simulink model "p4_individual_simulink"  (R2024b)
settings: Solver=VariableStepAuto  StartTime=0  StopTime=500  FixedStep=.1  RelTol=1e-3
values from neighbouring files (symbols this model uses):
  C0 = 0.0041    [p4_indiviual_init_cons.m]
  C1 = 0.000066    (= 6.6e-05)    [p4_indiviual_init_cons.m]
  C2 = 0.5*Rho*A*Cd    (= 0.5733)    [p4_indiviual_init_cons.m]
  efficency = .95    (= 0.95)    [p4_indiviual_init_cons.m]
undefined symbols (not defined in the file or in its folder): carData, datBat, datMotor
settings Model: Creator=Jake Sanders  LastModifiedBy=Jake Sanders

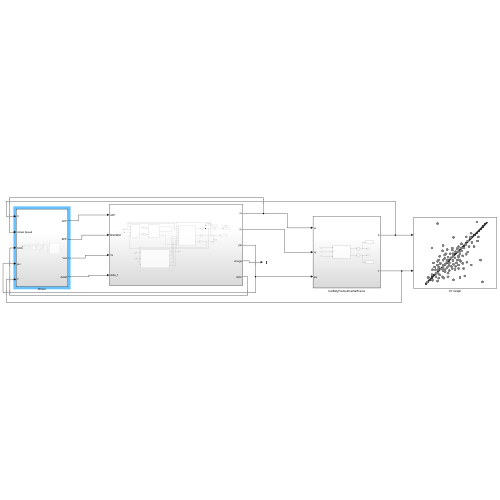
[thumbnail: Simulink's stored preview of the top-level diagram]
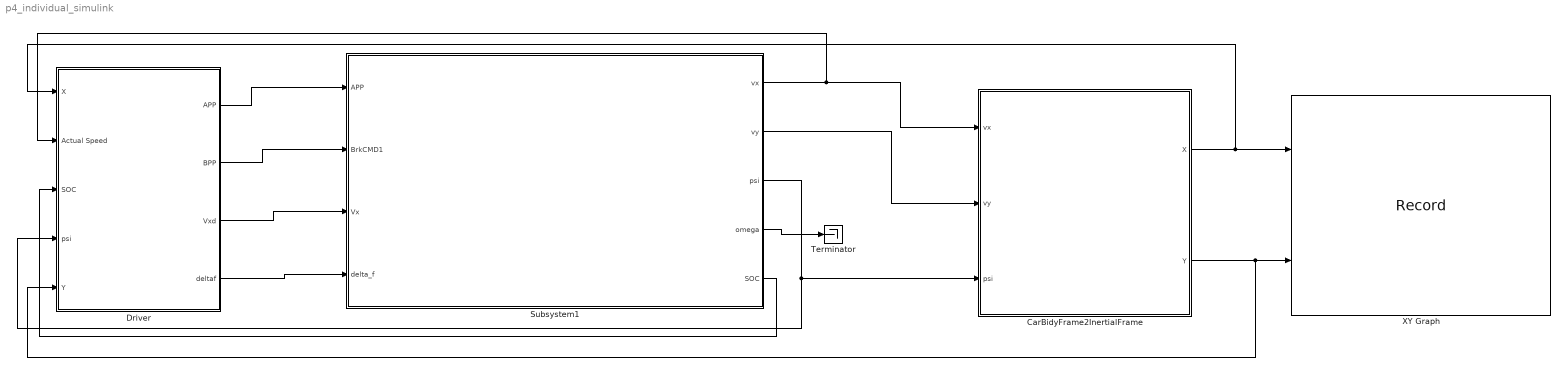
== system p4_individual_simulink ==
  CarBidyFrame2InertialFrame : Subsystem
  Driver : Subsystem
  Subsystem1 : Subsystem
  Terminator : Terminator
  XY Graph : Record  FileSettingsInternal="{\"entries\":[{\"content\":{\"excelSettings\":{\"content\":{},\"type\":\"Streamout.ExcelSettings\"}},\"type\":\"Streamout.FileSettingStorage\",\"uuid\":\"\"}],\"packageUris\":[\"http:\\/\\/schema.mathworks.com\\/mf0\\/streamout_blocks\\/R2020a\"],\"version\":\"1.0\"}"  Layout=[1 1]  SignalsInternal="{\"entries\":[{\"content\":{\"signals\":[{\"content\":{\"blockPath\":[],\"dimensions\":[1],\"domain\":\"\",\"lineColor\":\"#a2142f\",\"plots\":[ 1 ],\"port\":1,\"sid\":[\"\"],\"signalID\":1,\"signalName\":\"CarBidyFrame2InertialFrame:1\"},\"type\":\"RecordBlkView.Signal\",\"uuid\":\"\"},{\"content\":{\"blockPath\":[],\"dimensions\":[1],\"domain\":\"\",\"lineColor\":\"#139fff\",\"plots\":[ 1 ],\"port\":2,\"sid\":[\"\"],\"signalID\":2,\"signalName\":\"CarBidyFrame2InertialFrame:2\"},\"type\":\"RecordBlkView.Signal\",\"uuid\":\"\"},{\"content\":{\"blockPath\":[],\"dimensions\":[1],\"domain\":\"\",\"lineColor\":\"#ff6929\",\"lineWidth\":2,\"port\":1,\"sid\":[\"\"],\"signalID\":3,\"signalName\":\"Integrator\"},\"type\":\"RecordBlkView.Signal\",\"uuid\":\"\"},{\"content\":{\"blockPath\":[],\"dimensions\":[1],\"domain\":\"\",\"lineColor\":\"#b746ff\",\"lineWidth\":2,\"port\":1,\"sid\":[\"\"],\"signalID\":4,\"signalName\":\"Integrator1\"},\"type\":\"RecordBlkView.Signal\",\"uuid\":\"\"},{\"content\":{\"blockPath\":[],\"dimensions\":[1],\"domain\":\"\",\"lineColor\":\"#64d413\",\"lineWidth\":2,\"port\":1,\"sid\":[\"\"],\"signalID\":5,\"signalName\":\"MATLAB Function3\"},\"type\":\"RecordBlkView.Signal\",\"uuid\":\"\"},{\"content\":{\"blockPath\":[],\"dimensions\":[1],\"domain\":\"\",\"lineColor\":\"#ff13a6\",\"lineWidth\":2,\"port\":1,\"sid\":[\"\"],\"signalID\":6,\"signalName\":\"MATLAB Function5\"},\"type\":\"RecordBlkView.Signal\",\"uuid\":\"\"},{\"content\":{\"blockPath\":[],\"dimensions\":[1],\"domain\":\"\",\"lineColor\":\"#fe330a\",\"lineWidth\":2,\"port\":1,\"sid\":[\"\"],\"signalID\":7,\"signalName\":\"Integrator\"},\"type\":\"RecordBlkView.Signal\",\"uuid\":\"\"},{\"content\":{\"blockPath\":[],\"dimensions\":[1],\"domain\":\"\",\"lineColor\":\"#22b573\",\"lineWidth\":2,\"port\":1,\"sid\":[\"\"],\"signalID\":8,\"signalName\":\"Integrator1\"},\"type\":\"RecordBlkView.Signal\",\"uuid\":\"\"},{\"content\":{\"blockPath\":[],\"dimensions\":[1],\"domain\":\"\",\"lineColor\":\"#0072bd\",\"lineWidth\":2,\"port\":1,\"sid\":[\"\"],\"signalID\":9,\"signalName\":\"Integrator2\"},\"type\":\"RecordBlkView.Signal\",\"uuid\":\"\"},{\"content\":{\"blockPath\":[],\"dimensions\":[1],\"domain\":\"\",\"lineColor\":\"#d95319\",\"lineWidth\":2,\"port\":1,\"sid\":[\"\"],\"signalID\":10,\"signalName\":\"drag forces\"},\"type\":\"RecordBlkView.Signal\",\"uuid\":\"\"},{\"content\":{\"blockPath\":[],\"dimensions\":[1],\"domain\":\"\",\"lineColor\":\"#edb120\",\"lineWidth\":2,\"port\":1,\"sid\":[\"\"],\"signalID\":11,\"signalName\":\"Electric Motor Drve:3\"},\"type\":\"RecordBlkView.Signal\",\"uuid\":\"\"},{\"content\":{\"blockPath\":[],\"dimensions\":[1],\"domain\":\"\",\"lineColor\":\"#7e2f8e\",\"lineWidth\":2,\"port\":1,\"sid\":[\"\"],\"signalID\":12,\"signalName\":\"Gain5\"},\"type\":\"RecordBlkView.Signal\",\"uuid\":\"\"},{\"content\":{\"blockPath\":[],\"dimensions\":[1],\"domain\":\"\",\"lineColor\":\"#77ac30\",\"lineWidth\":2,\"port\":1,\"sid\":[\"\"],\"signalID\":13,\"signalName\":\"Integrator1\"},\"type\":\"RecordBlkView.Signal\",\"uuid\":\"\"},{\"content\":{\"blockPath\":[],\"dimensions\":[1],\"domain\":\"\",\"lineColor\":\"#4dbeee\",\"lineWidth\":2,\"port\":1,\"sid\":[\"\"],\"signalID\":14,\"signalName\":\"1-D Lookup\\nTable\"},\"type\":\"RecordBlkView.Signal\",\"uuid\":\"\"},{\"content\":{\"blockPath\":[],\"dimensions\":[1],\"domain\":\"\",\"lineColor\":\"#a2142f\",\"lineWidth\":2,\"port\":1,\"sid\":[\"\"],\"signalID\":15,\"signalName\":\"Motor Efficiency Table\"},\"type\":\"RecordBlkView.Signal\",\"uuid\":\"\"},{\"content\":{\"blockPath\":[],\"dimensions\":[1],\"domain\":\"\",\"lineColor\":\"#139fff\",\"lineWidth\":2,\"port\":1,\"sid\":[\"\"],\"signalID\":16,\"signalName\":\"Product1\"},\"type\":\"RecordBlkView.Signal\",\"uuid\":\"\"},{\"content\":{\"blockPath\":[],\"dimensions\":[1],\"domain\":\"\",\"lineColor\":\"#ff6929\",\"lineWidth\":2,\"port\":1,\"sid\":[\"\"],\"signalID\":17,\"signalName\":\"Integrator\"},\"type\":\"RecordBlkView.Signal\",\"uuid\":\"\"},{\"content\":{\"blockPath\":[],\"dimensions\":[1],\"domain\":\"\",\"lineColor\":\"#b746ff\",\"lineWidth\":2,\"port\":1,\"sid\":[\"\"],\"signalID\":18,\"signalName\":\"Bus Voltage\"},\"type\":\"RecordBlkView.Signal\",\"uuid\":\"\"},{\"content\":{\"blockPath\":[],\"dimensions\":[1],\"domain\":\"\",\"lineColor\":\"#64d413\",\"lineWidth\":2,\"port\":1,\"sid\":[\"\"],\"signalID\":19,\"signalName\":\"Unit Delay\"},\"type\":\"RecordBlkView.Signal\",\"uuid\":\"\"},{\"content\":{\"blockPath\":[],\"dimensions\":[1],\"domain\":\"\",\"lineColor\":\"#ff13a6\",\"lineWidth\":2,\"port\":1,\"sid\":[\"\"],\"signalID\":20,\"signalName\":\"MATLAB Function:2\"},\"type\":\"RecordBlkView.Signal\",\"uuid\":\"\"}]},\"type\":\"RecordBlkView.InputSignals\",\"uuid\":\"\"}],\"packageUris\":[\"http:\\/\\/schema.mathworks.com\\/mf0\\/streamout_blocks\\/R2020a\"],\"version\":\"1.0\"}"  VisualizationBindings="{\"xyplotplugin\":{\"info\":[{\"series\":[{\"bindingParametersList\":[{\"parameter\":\"X-Axis\",\"signalID\":1,\"signalName\":\"CarBidyFrame2InertialFrame:1\"},{\"parameter\":\"Y-Axis\",\"signalID\":2,\"signalName\":\"CarBidyFrame2InertialFrame:2\"}],\"seriesID\":0}],\"subplotID\":1}]}}"  CompatibilityTag=XY
  wires:
  CarBidyFrame2InertialFrame/2(Y) -> Driver/5(Y), XY Graph/2
  CarBidyFrame2InertialFrame/1(X) -> Driver/1(X), XY Graph/1
  Driver/1(APP) -> Subsystem1/1(APP)
  Driver/2(BPP) -> Subsystem1/2(BrkCMD1)
  Driver/3(Vxd) -> Subsystem1/3(Vx)
  Driver/4(deltaf) -> Subsystem1/4(delta_f)
  Subsystem1/5(SOC) -> Driver/3(SOC)
  Subsystem1/3(psi) -> Driver/4(psi), CarBidyFrame2InertialFrame/3(psi)
  Subsystem1/2(vy) -> CarBidyFrame2InertialFrame/2(vy)
  Subsystem1/1(vx) -> Driver/2(Actual Speed), CarBidyFrame2InertialFrame/1(vx)
  Subsystem1/4(omega) -> Terminator/1

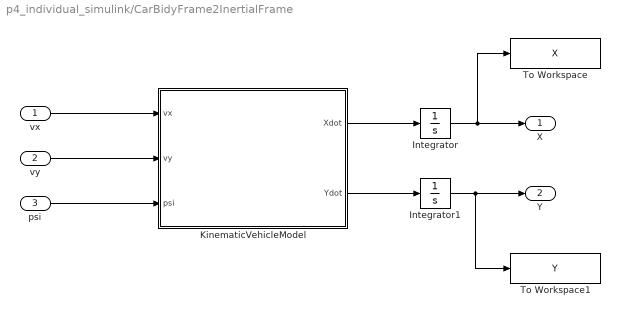
== system p4_individual_simulink/CarBidyFrame2InertialFrame ==
  vx : Inport
  vy : Inport  Port=2
  psi : Inport  Port=3
  Integrator : Integrator  InitialCondition=carData.init.X0
  Integrator1 : Integrator  InitialCondition=carData.init.Y0
  KinematicVehicleModel : MATLAB Function  TreatAsAtomicUnit=on
  To Workspace : ToWorkspace  VariableName=X  SaveFormat=Timeseries  SampleTime=.5
  To Workspace1 : ToWorkspace  VariableName=Y  SaveFormat=Timeseries  SampleTime=.5
  X : Outport
  Y : Outport  Port=2
  wires:
  vy/1 -> KinematicVehicleModel/2(vy)
  vx/1 -> KinematicVehicleModel/1(vx)
  psi/1 -> KinematicVehicleModel/3(psi)
  KinematicVehicleModel/1(Xdot) -> Integrator/1
  KinematicVehicleModel/2(Ydot) -> Integrator1/1
  Integrator/1 -> To Workspace/1, X/1
  Integrator1/1 -> To Workspace1/1, Y/1

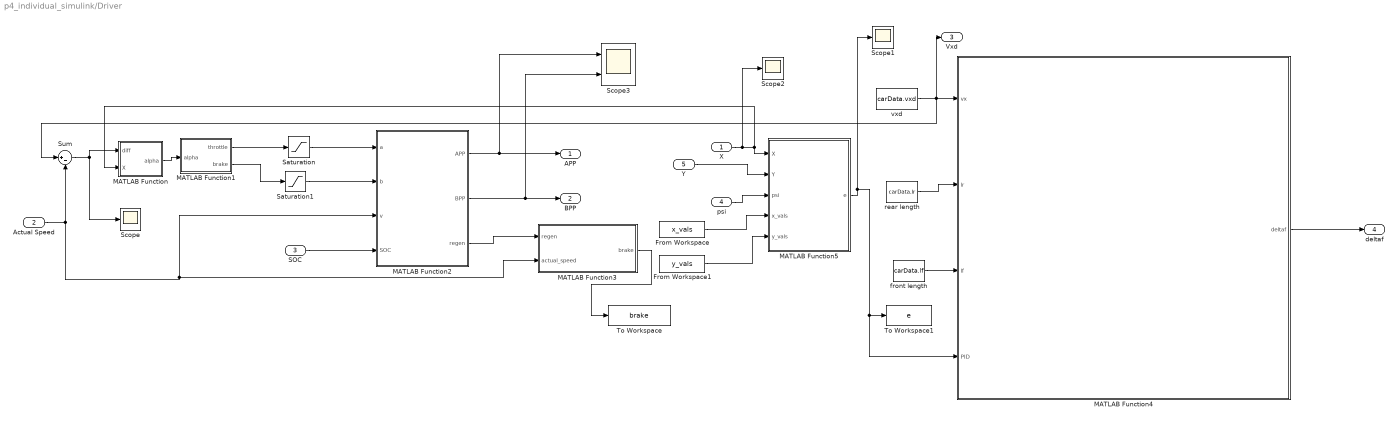
== system p4_individual_simulink/Driver ==
  X : Inport
  Actual Speed : Inport  Port=2
  SOC : Inport  Port=3
  psi : Inport  Port=4
  Y : Inport  Port=5
  From Workspace : FromWorkspace  VariableName=x_vals
  From Workspace1 : FromWorkspace  VariableName=y_vals
  MATLAB Function : MATLAB Function  TreatAsAtomicUnit=on
  MATLAB Function1 : MATLAB Function  TreatAsAtomicUnit=on
  MATLAB Function2 : MATLAB Function  TreatAsAtomicUnit=on
  MATLAB Function3 : MATLAB Function  TreatAsAtomicUnit=on
  MATLAB Function4 : MATLAB Function  TreatAsAtomicUnit=on
  MATLAB Function5 : MATLAB Function  TreatAsAtomicUnit=on
  Saturation : Saturate  UpperLimit=1  LowerLimit=0
  Saturation1 : Saturate  UpperLimit=0  LowerLimit=-1
  Scope : Scope
  Scope1 : Scope
  Scope2 : Scope
  Scope3 : Scope  NumInputPorts=2
  Sum : Sum  Inputs=|+-
  To Workspace : ToWorkspace  VariableName=brake  SaveFormat=Timeseries  SampleTime=-1
  To Workspace1 : ToWorkspace  VariableName=e  SaveFormat=Timeseries  SampleTime=-1
  front length : Constant  Value=carData.lf
  rear length : Constant  Value=carData.lr
  vxd : Constant  Value=carData.vxd
  APP : Outport
  BPP : Outport  Port=2
  Vxd : Outport  Port=3
  deltaf : Outport  Port=4
  wires:
  Actual Speed/1 -> Sum/2, MATLAB Function2/3(v), MATLAB Function3/2(actual_speed)
  MATLAB Function/1(alpha) -> MATLAB Function1/1(alpha)
  Sum/1 -> Scope/1, MATLAB Function/1(diff)
  Saturation/1 -> MATLAB Function2/1(a)
  MATLAB Function2/2(BPP) -> Scope3/2, BPP/1
  MATLAB Function1/1(throttle) -> Saturation/1
  MATLAB Function2/1(APP) -> Scope3/1, APP/1
  MATLAB Function2/3(regen) -> MATLAB Function3/1(regen)
  MATLAB Function3/1(brake) -> To Workspace/1
  MATLAB Function1/2(brake) -> Saturation1/1
  Saturation1/1 -> MATLAB Function2/2(b)
  SOC/1 -> MATLAB Function2/4(SOC)
  X/1 -> Scope2/1, MATLAB Function5/1(X), MATLAB Function/2(X)
  MATLAB Function5/1(e) -> Scope1/1, MATLAB Function4/4(PID), To Workspace1/1
  Y/1 -> MATLAB Function5/2(Y)
  front length/1 -> MATLAB Function4/3(lf)
  psi/1 -> MATLAB Function5/3(psi)
  vxd/1 -> Sum/1, Vxd/1, MATLAB Function4/1(vx)
  rear length/1 -> MATLAB Function4/2(lr)
  MATLAB Function4/1(deltaf) -> deltaf/1
  From Workspace/1 -> MATLAB Function5/4(x_vals)
  From Workspace1/1 -> MATLAB Function5/5(y_vals)

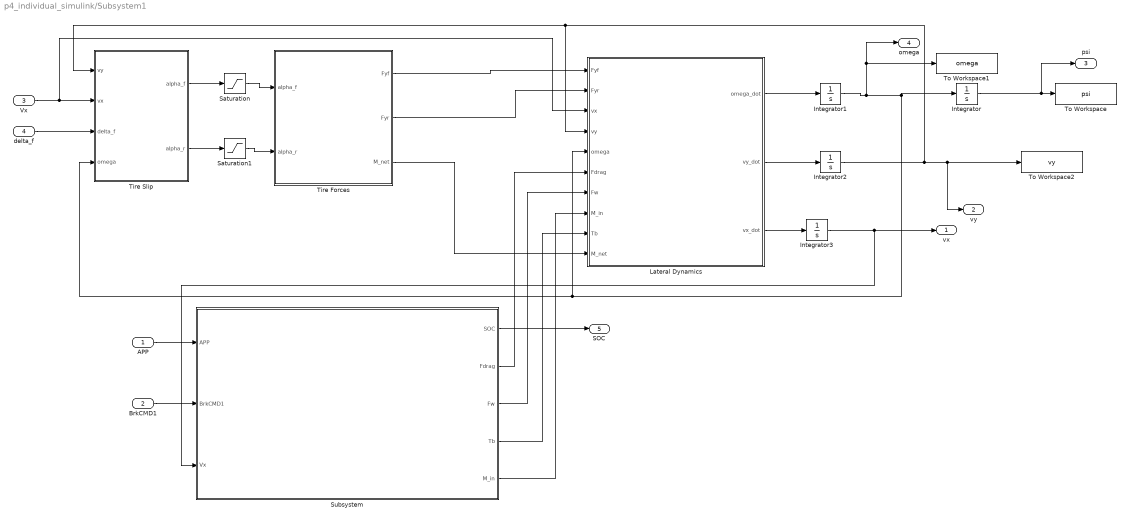
== system p4_individual_simulink/Subsystem1 ==
  APP : Inport
  BrkCMD1 : Inport  Port=2
  Vx : Inport  Port=3
  delta_f : Inport  Port=4
  " Tire Slip" : MATLAB Function  TreatAsAtomicUnit=on
  Integrator : Integrator  InitialCondition=carData.init.psi0
  Integrator1 : Integrator  InitialCondition=carData.init.omega0
  Integrator2 : Integrator  InitialCondition=carData.init.vy0
  Integrator3 : Integrator
  Lateral Dynamics : MATLAB Function  TreatAsAtomicUnit=on
  Saturation : Saturate
  Saturation1 : Saturate
  Subsystem : Subsystem
  Tire Forces : MATLAB Function  TreatAsAtomicUnit=on
  To Workspace : ToWorkspace  VariableName=psi  SaveFormat=Timeseries  SampleTime=.5
  To Workspace1 : ToWorkspace  VariableName=omega  SaveFormat=Timeseries  SampleTime=-1
  To Workspace2 : ToWorkspace  VariableName=vy  SaveFormat=Timeseries  SampleTime=-1
  vx : Outport
  vy : Outport  Port=2
  psi : Outport  Port=3
  omega : Outport  Port=4
  SOC : Outport  Port=5
  wires:
  APP/1 -> Subsystem/1(APP)
  BrkCMD1/1 -> Subsystem/2(BrkCMD1)
  Subsystem/1(SOC) -> SOC/1
  Lateral Dynamics/1(omega_dot) -> Integrator1/1
  Integrator2/1 -> Lateral Dynamics/4(vy), " Tire Slip"/1(vy), To Workspace2/1, vy/1
  Integrator1/1 -> Lateral Dynamics/5(omega), " Tire Slip"/4(omega), Integrator/1, omega/1, To Workspace1/1
  Saturation/1 -> Tire Forces/1(alpha_f)
  Tire Forces/1(Fyf) -> Lateral Dynamics/1(Fyf)
  Saturation1/1 -> Tire Forces/2(alpha_r)
  delta_f/1 -> " Tire Slip"/3(delta_f)
  Lateral Dynamics/2(vy_dot) -> Integrator2/1
  " Tire Slip"/1(alpha_f) -> Saturation/1
  Integrator/1 -> psi/1, To Workspace/1
  " Tire Slip"/2(alpha_r) -> Saturation1/1
  Tire Forces/2(Fyr) -> Lateral Dynamics/2(Fyr)
  Vx/1 -> Lateral Dynamics/3(vx), " Tire Slip"/2(vx)
  Tire Forces/3(M_net) -> Lateral Dynamics/10(M_net)
  Subsystem/2(Fdrag) -> Lateral Dynamics/6(Fdrag)
  Subsystem/3(Fw) -> Lateral Dynamics/7(Fw)
  Subsystem/4(Tb) -> Lateral Dynamics/9(Tb)
  Subsystem/5(M_in) -> Lateral Dynamics/8(M_in)
  Lateral Dynamics/3(vx_dot) -> Integrator3/1
  Integrator3/1 -> Subsystem/3(Vx), vx/1

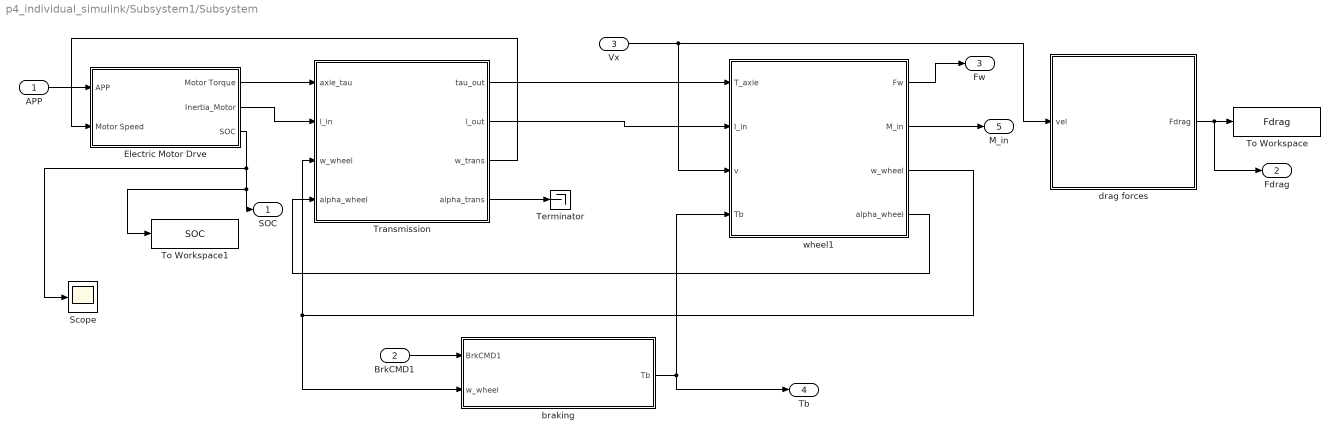
== system p4_individual_simulink/Subsystem1/Subsystem ==
  APP : Inport
  BrkCMD1 : Inport  Port=2
  Vx : Inport  Port=3
  Electric Motor Drve : Subsystem
  Scope : Scope
  Terminator : Terminator
  To Workspace : ToWorkspace  VariableName=Fdrag  SaveFormat=Timeseries  SampleTime=-1
  To Workspace1 : ToWorkspace  VariableName=SOC  SaveFormat=Timeseries  SampleTime=-1
  Transmission : Subsystem
  braking : Subsystem
  drag forces : Subsystem
  wheel1 : Subsystem
  SOC : Outport
  Fdrag : Outport  Port=2
  Fw : Outport  Port=3
  Tb : Outport  Port=4
  M_in : Outport  Port=5
  wires:
  Transmission/1(tau_out) -> wheel1/1(T_axle)
  Transmission/3(w_trans) -> Electric Motor Drve/2(Motor Speed)
  wheel1/4(alpha_wheel) -> Transmission/4(alpha_wheel)
  Electric Motor Drve/2(Inertia_Motor) -> Transmission/2(l_in)
  Electric Motor Drve/1(Motor Torque) -> Transmission/1(axle_tau)
  wheel1/3(w_wheel) -> Transmission/3(w_wheel), braking/2(w_wheel)
  Electric Motor Drve/3(SOC) -> Scope/1, To Workspace1/1, SOC/1
  APP/1 -> Electric Motor Drve/1(APP)
  BrkCMD1/1 -> braking/1(BrkCMD1)
  drag forces/1(Fdrag) -> Fdrag/1, To Workspace/1
  wheel1/1(Fw) -> Fw/1
  braking/1(Tb) -> wheel1/4(Tb), Tb/1
  Vx/1 -> wheel1/3(v), drag forces/1(vel)
  wheel1/2(M_in) -> M_in/1
  Transmission/2(l_out) -> wheel1/2(I_in)
  Transmission/4(alpha_trans) -> Terminator/1

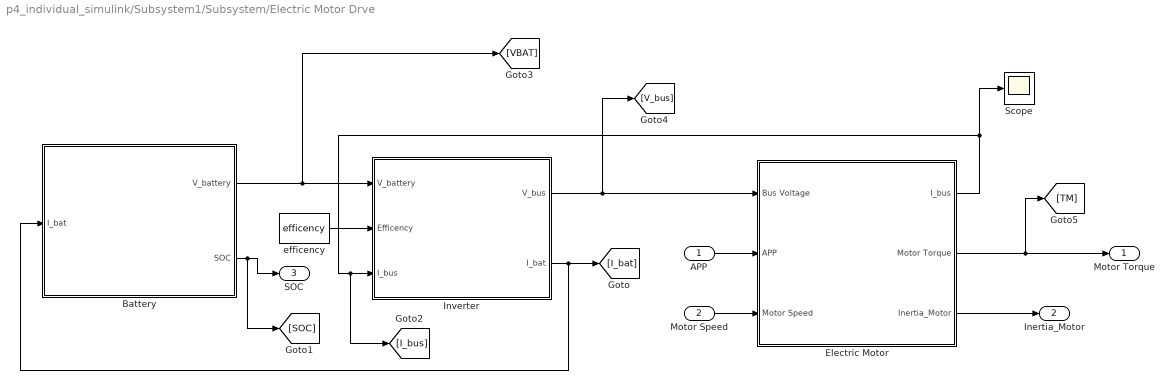
== system p4_individual_simulink/Subsystem1/Subsystem/Electric Motor Drve ==
  APP : Inport
  Motor Speed : Inport  Port=2
  Battery : Subsystem
  Electric Motor : Subsystem
  Inverter : Subsystem
  Scope : Scope
  efficency : Constant  Value=efficency
  Motor Torque : Outport
  Inertia_Motor : Outport  Port=2
  SOC : Outport  Port=3
  wires:
  Inverter/1(V_bus) -> [V_bus], Electric Motor/1(Bus Voltage)
  Inverter/2(I_bat) -> Battery/1(I_bat), [I_bat]
  Electric Motor/1(I_bus) -> Scope/1, [I_bus], Inverter/3(I_bus)
  Electric Motor/2(Motor Torque) -> [TM], Motor Torque/1
  Electric Motor/3(Inertia_Motor) -> Inertia_Motor/1
  APP/1 -> Electric Motor/2(APP)
  Motor Speed/1 -> Electric Motor/3(Motor Speed)
  efficency/1 -> Inverter/2(Efficency)
  Battery/1(V_battery) -> [VBAT], Inverter/1(V_battery)
  Battery/2(SOC) -> [SOC], SOC/1

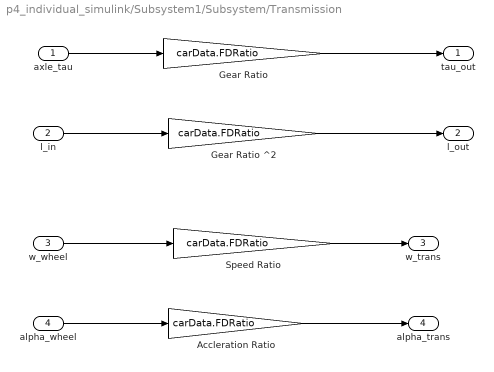
== system p4_individual_simulink/Subsystem1/Subsystem/Transmission ==
  axle_tau : Inport
  l_in : Inport  Port=2
  w_wheel : Inport  Port=3
  alpha_wheel : Inport  Port=4
  Accleration Ratio : Gain  Gain=carData.FDRatio
  Gear Ratio : Gain  Gain=carData.FDRatio
  Gear Ratio ^2 : Gain  Gain=carData.FDRatio
  Speed Ratio : Gain  Gain=carData.FDRatio
  tau_out : Outport
  l_out : Outport  Port=2
  w_trans : Outport  Port=3
  alpha_trans : Outport  Port=4
  wires:
  axle_tau/1 -> Gear Ratio/1
  Gear Ratio/1 -> tau_out/1
  w_wheel/1 -> Speed Ratio/1
  Speed Ratio/1 -> w_trans/1
  alpha_wheel/1 -> Accleration Ratio/1
  Accleration Ratio/1 -> alpha_trans/1
  l_in/1 -> Gear Ratio ^2/1
  Gear Ratio ^2/1 -> l_out/1

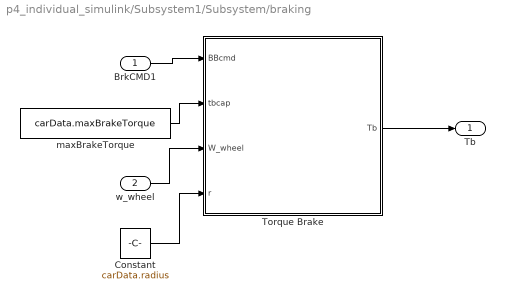
== system p4_individual_simulink/Subsystem1/Subsystem/braking ==
  BrkCMD1 : Inport
  w_wheel : Inport  Port=2
  Constant : Constant  Value=carData.radius
  Torque Brake : MATLAB Function  TreatAsAtomicUnit=on
  maxBrakeTorque : Constant  Value=carData.maxBrakeTorque
  Tb : Outport
  wires:
  w_wheel/1 -> Torque Brake/3(W_wheel)
  maxBrakeTorque/1 -> Torque Brake/2(tbcap)
  Torque Brake/1(Tb) -> Tb/1
  BrkCMD1/1 -> Torque Brake/1(BBcmd)
  Constant/1 -> Torque Brake/4(r)

== system p4_individual_simulink/Subsystem1/Subsystem/drag forces ==
  vel : Inport
  C0 : Constant  Value=C0
  C1 : Constant  Value=C1
  C2 : Constant  Value=C2
  MATLAB Function1 : MATLAB Function  TreatAsAtomicUnit=on
  Fdrag : Outport
  wires:
  vel/1 -> MATLAB Function1/1(vel)
  C0/1 -> MATLAB Function1/2(C0)
  C1/1 -> MATLAB Function1/3(C1)
  C2/1 -> MATLAB Function1/4(C2)
  MATLAB Function1/1(Fdrag) -> Fdrag/1

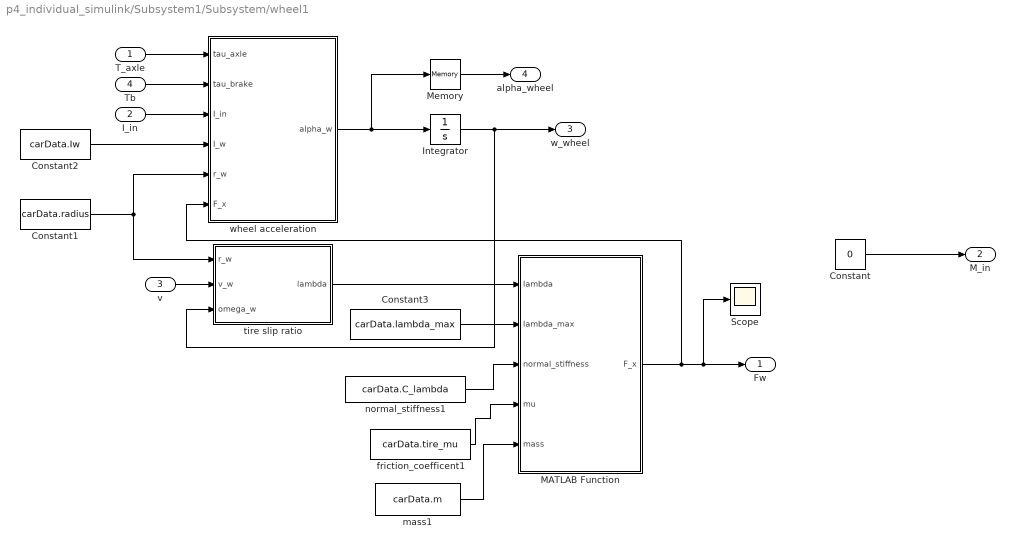
== system p4_individual_simulink/Subsystem1/Subsystem/wheel1 ==
  T_axle : Inport
  I_in : Inport  Port=2
  v : Inport  Port=3
  Tb : Inport  Port=4
  Constant : Constant  Value=0
  Constant1 : Constant  Value=carData.radius
  Constant2 : Constant  Value=carData.Iw
  Constant3 : Constant  Value=carData.lambda_max
  Integrator : Integrator
  MATLAB Function : MATLAB Function  TreatAsAtomicUnit=on
  Memory : Memory
  Scope : Scope
  friction_coefficent1 : Constant  Value=carData.tire_mu
  mass1 : Constant  Value=carData.m
  normal_stiffness1 : Constant  Value=carData.C_lambda
  tire slip ratio : MATLAB Function  TreatAsAtomicUnit=on
  wheel acceleration : MATLAB Function  TreatAsAtomicUnit=on
  Fw : Outport
  M_in : Outport  Port=2
  w_wheel : Outport  Port=3
  alpha_wheel : Outport  Port=4
  wires:
  MATLAB Function/1(F_x) -> wheel acceleration/6(F_x), Scope/1, Fw/1
  normal_stiffness1/1 -> MATLAB Function/3(normal_stiffness)
  friction_coefficent1/1 -> MATLAB Function/4(mu)
  mass1/1 -> MATLAB Function/5(mass)
  Constant3/1 -> MATLAB Function/2(lambda_max)
  tire slip ratio/1(lambda) -> MATLAB Function/1(lambda)
  Constant/1 -> M_in/1
  Memory/1 -> alpha_wheel/1
  wheel acceleration/1(alpha_w) -> Integrator/1, Memory/1
  Constant1/1 -> tire slip ratio/1(r_w), wheel acceleration/5(r_w)
  Constant2/1 -> wheel acceleration/4(I_w)
  I_in/1 -> wheel acceleration/3(I_in)
  Tb/1 -> wheel acceleration/2(tau_brake)
  T_axle/1 -> wheel acceleration/1(tau_axle)
  Integrator/1 -> w_wheel/1, tire slip ratio/3(omega_w)
  v/1 -> tire slip ratio/2(v_w)

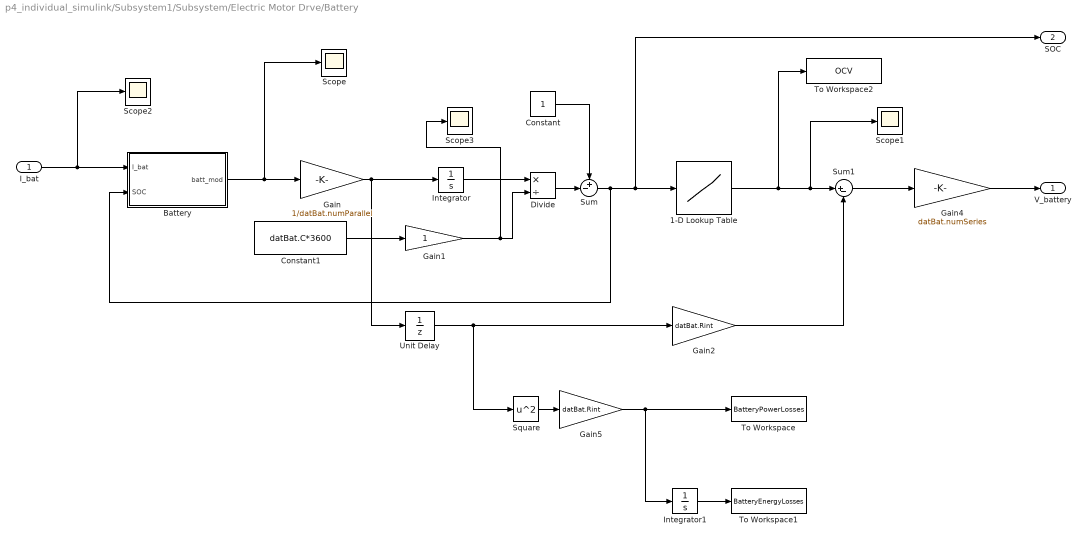
== system p4_individual_simulink/Subsystem1/Subsystem/Electric Motor Drve/Battery ==
  I_bat : Inport
  1-D Lookup Table : Lookup_n-D  NumberOfTableDimensions=1  BreakpointsForDimension1=datBat.SOC  Table=datBat.OCV  InternalRulePriority=Speed  RndMeth=Simplest
  Battery : MATLAB Function  TreatAsAtomicUnit=on
  Constant : Constant
  Constant1 : Constant  Value=datBat.C*3600
  Divide : Product  Inputs=*/
  Gain : Gain  Gain=1/datBat.numParallel
  Gain1 : Gain
  Gain2 : Gain  Gain=datBat.Rint
  Gain4 : Gain  Gain=datBat.numSeries
  Gain5 : Gain  Gain=datBat.Rint
  Integrator : Integrator
  Integrator1 : Integrator
  Scope{,1..3} (4 alike) : Scope
  Square : Math  Operator=square
  Sum : Sum  Inputs=+-|
  Sum1 : Sum  Inputs=|+-
  To Workspace : ToWorkspace  VariableName=BatteryPowerLosses  SaveFormat=Timeseries  SampleTime=-1
  To Workspace1 : ToWorkspace  VariableName=BatteryEnergyLosses  SaveFormat=Timeseries  SampleTime=-1
  To Workspace2 : ToWorkspace  VariableName=OCV  SaveFormat=Timeseries  SampleTime=-1
  Unit Delay : UnitDelay  SampleTime=-1  HasFrameUpgradeWarning=on
  V_battery : Outport
  SOC : Outport  Port=2
  wires:
  Gain5/1 -> Integrator1/1, To Workspace/1
  Integrator/1 -> Divide/1
  1-D Lookup Table/1 -> To Workspace2/1, Scope1/1, Sum1/1
  Sum1/1 -> Gain4/1
  Gain2/1 -> Sum1/2
  Battery/1(batt_mod) -> Scope/1, Gain/1
  Sum/1 -> Battery/2(SOC), SOC/1, 1-D Lookup Table/1
  Unit Delay/1 -> Square/1, Gain2/1
  Constant/1 -> Sum/1
  Divide/1 -> Sum/2
  Constant1/1 -> Gain1/1
  Integrator1/1 -> To Workspace1/1
  Gain4/1 -> V_battery/1
  Square/1 -> Gain5/1
  Gain1/1 -> Scope3/1, Divide/2
  I_bat/1 -> Scope2/1, Battery/1(I_bat)
  Gain/1 -> Unit Delay/1, Integrator/1

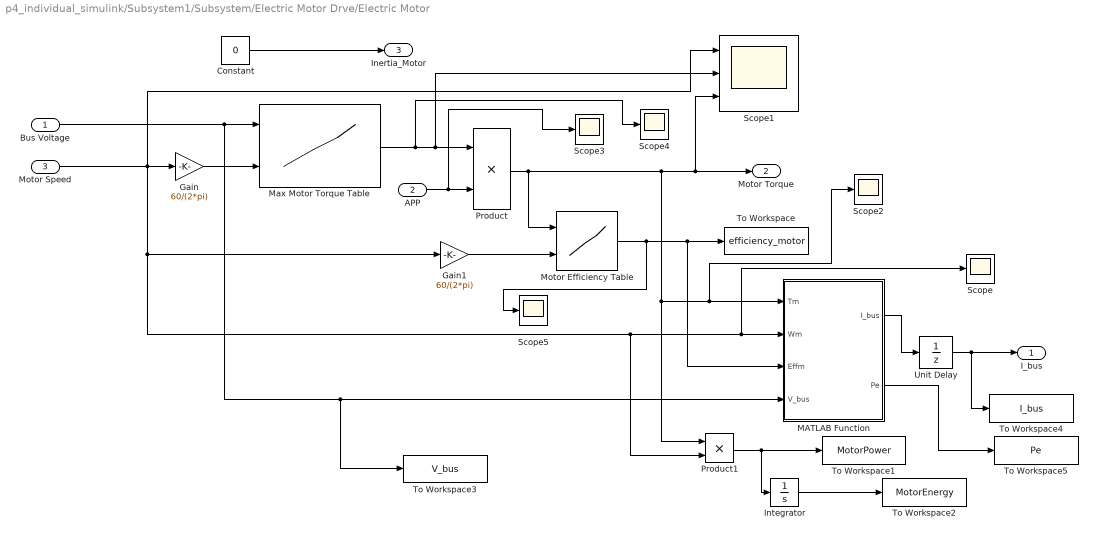
== system p4_individual_simulink/Subsystem1/Subsystem/Electric Motor Drve/Electric Motor ==
  Bus Voltage : Inport
  APP : Inport  Port=2
  Motor Speed : Inport  Port=3
  Constant : Constant  Value=0
  Gain : Gain  Gain=60/(2*pi)
  Gain1 : Gain  Gain=60/(2*pi)
  Integrator : Integrator
  MATLAB Function : MATLAB Function  TreatAsAtomicUnit=on
  "Max Motor Torque Table " : Lookup_n-D  BreakpointsForDimension1=datMotor.vbus  BreakpointsForDimension2=datMotor.rpm  Table=datMotor.maxtorque  InternalRulePriority=Speed  RndMeth=Simplest
      settings: InputPortMap=u0,u1
  Motor Efficiency Table : Lookup_n-D  BreakpointsForDimension1=datMotor.eta_torque  BreakpointsForDimension2=datMotor.eta_speed  Table=datMotor.eta_val  InternalRulePriority=Speed  RndMeth=Simplest
      settings: InputPortMap=u0,u1
  Product : Product
  Product1 : Product
  Scope{,2..5} (5 alike) : Scope
  Scope1 : Scope  NumInputPorts=3
  To Workspace : ToWorkspace  VariableName=efficiency_motor  SaveFormat=Timeseries  SampleTime=-1
  To Workspace1 : ToWorkspace  VariableName=MotorPower  SaveFormat=Timeseries  SampleTime=-1
  To Workspace2 : ToWorkspace  VariableName=MotorEnergy  SaveFormat=Timeseries  SampleTime=.5
  To Workspace3 : ToWorkspace  VariableName=V_bus  SaveFormat=Timeseries  SampleTime=-1
  To Workspace4 : ToWorkspace  VariableName=I_bus  SaveFormat=Timeseries  SampleTime=-1
  To Workspace5 : ToWorkspace  VariableName=Pe  SaveFormat=Timeseries  SampleTime=-1
  Unit Delay : UnitDelay  SampleTime=-1  HasFrameUpgradeWarning=on
  I_bus : Outport
  Motor Torque : Outport  Port=2
  Inertia_Motor : Outport  Port=3
  wires:
  Motor Speed/1 -> Gain1/1, Scope/1, MATLAB Function/2(Wm), Product1/2, Gain/1, Scope1/1
  Gain/1 -> "Max Motor Torque Table "/2
  Bus Voltage/1 -> "Max Motor Torque Table "/1, To Workspace3/1, MATLAB Function/4(V_bus)
  "Max Motor Torque Table "/1 -> Scope4/1, Product/1, Scope1/2
  APP/1 -> Scope3/1, Product/2
  Gain1/1 -> Motor Efficiency Table/2
  Product/1 -> Scope1/3, Motor Torque/1, Scope2/1, MATLAB Function/1(Tm), Product1/1, Motor Efficiency Table/1
  Constant/1 -> Inertia_Motor/1
  Motor Efficiency Table/1 -> Scope5/1, MATLAB Function/3(Effm), To Workspace/1
  Product1/1 -> Integrator/1, To Workspace1/1
  Integrator/1 -> To Workspace2/1
  MATLAB Function/1(I_bus) -> Unit Delay/1
  Unit Delay/1 -> I_bus/1, To Workspace4/1
  MATLAB Function/2(Pe) -> To Workspace5/1

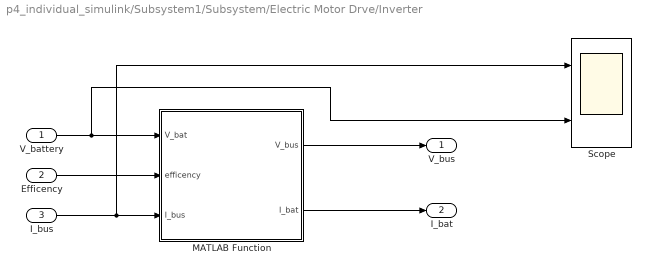
== system p4_individual_simulink/Subsystem1/Subsystem/Electric Motor Drve/Inverter ==
  V_battery : Inport
  Efficency : Inport  Port=2
  I_bus : Inport  Port=3
  MATLAB Function : MATLAB Function  TreatAsAtomicUnit=on
  Scope : Scope  NumInputPorts=2
  V_bus : Outport
  I_bat : Outport  Port=2
  wires:
  V_battery/1 -> Scope/2, MATLAB Function/1(V_bat)
  Efficency/1 -> MATLAB Function/2(efficency)
  I_bus/1 -> Scope/1, MATLAB Function/3(I_bus)
  MATLAB Function/1(V_bus) -> V_bus/1
  MATLAB Function/2(I_bat) -> I_bat/1

== matlab function p4_individual_simulink/Subsystem1/ Tire Slip ==
  data: vy input; alpha_f output; vx input; delta_f input; omega input; alpha_r output; carData parameter
function [alpha_f, alpha_r] = fcn(vy, vx, delta_f, omega, carData)

if abs(vx) > 0
    alpha_f = delta_f - (vy + omega * carData.lf) / vx;
    alpha_r = - (vy - omega * carData.lr) / vx;
else
    alpha_f = 0;
    alpha_r = 0;
end
end

== matlab function p4_individual_simulink/Subsystem1/Subsystem/Electric Motor Drve/Inverter/MATLAB Function ==
  data: V_bat input; V_bus output; I_bat output; efficency input; I_bus input
function [V_bus, I_bat] = fcn(V_bat, efficency, I_bus)
    
    V_bus = V_bat;
    P_bus = V_bus*I_bus;
    sgn_Pbus = P_bus / (abs(P_bus)+0.001);

    if V_bat > 1
        I_bat = (P_bus / efficency^sgn_Pbus) / V_bat;
    else
        I_bat = 0;
    end
end

== matlab function p4_individual_simulink/Subsystem1/Lateral Dynamics ==
  data: omega_dot output; Fyf input; Fyr input; vx input; vy input; vy_dot output; omega input; carData parameter; Fdrag input; Fw input; M_in input; Tb input; vx_dot output; M_net input
function [omega_dot, vy_dot, vx_dot] = fcn(Fyf, Fyr, vx, vy, omega, carData, Fdrag, Fw, M_in, Tb, M_net)

Fy = Fyf + Fyr;
vy_dot = (Fy / carData.m) - omega * vx;

M = Fyf * carData.lf - Fyr * carData.lr;

Fb = Tb/carData.radius;

vx_dot = (Fw-Fb-Fdrag)/(M_in+carData.m) + vy*omega;

omega_dot = M_net / carData.I;
end

== matlab function p4_individual_simulink/Subsystem1/Tire Forces ==
  data: alpha_f input; Fyf output; alpha_r input; Fyr output; carData parameter; M_net output
function [Fyf, Fyr, M_net] = fcn(alpha_f, alpha_r, carData)

Fyf = min(carData.Fyfmax, carData.Calpha_f * alpha_f);
Fyr = min(carData.Fyrmax, carData.Calpha_r * alpha_r);

M_net = (Fyf*carData.lf) - (Fyr*carData.lr);
end

== matlab function p4_individual_simulink/Driver/MATLAB Function2 ==
  data: a input; APP output; b input; v input; SOC input; BPP output; regen output
function [APP, BPP, regen] = fcn(a, b, v, SOC)

    speed1 = 5*(1600/3200);
    speed2 = 25*(1600/3200);
    speed_diff = speed2 - speed1; 

    absV = abs(v);

    if absV < speed1
        regen = 0;
    elseif absV <= speed2
        regen = 0.95 * (absV - speed1)/speed_diff;
    else
        regen = 0.95;
    end

    if SOC < 0.8
        SOCfactor = 1;
    elseif SOC < 1
        SOCfactor = 1 - (SOC - 0.8)/(1-0.8);
    else
        SOCfactor = 0;
    end

    regen = regen * SOCfactor;

    APP = a + b * regen;
    BPP = b * (1 - regen);

== matlab function p4_individual_simulink/Subsystem1/Subsystem/braking/Torque Brake ==
  data: BBcmd input; tbcap input; Tb output; W_wheel input; r input
function Tb =fcn(BBcmd,tbcap, W_wheel, r)

Tb = -BBcmd * tbcap * (W_wheel / (abs(W_wheel)+ .001));

end

== matlab function p4_individual_simulink/Subsystem1/Subsystem/drag forces/MATLAB Function1 ==
  data: vel input; Fdrag output; C0 input; C1 input; C2 input
function Fdrag = fcn(vel, C0, C1, C2)

Fdrag = C0 + C1*vel + C2*(vel^2);

== matlab function p4_individual_simulink/Subsystem1/Subsystem/wheel1/tire slip ratio ==
  data: r_w input; v_w input; lambda output; omega_w input
function lambda = tire_slip_ratio(r_w, v_w,omega_w)

epsillon = 0.0001; %small num for numerical smootening

if (r_w * omega_w >= v_w - epsillon)
    lambda = (r_w * omega_w - v_w)/ (abs(r_w*omega_w)+epsillon);
else
    lambda = (r_w * omega_w - v_w)/ (abs(v_w)+epsillon);
end

== matlab function p4_individual_simulink/Subsystem1/Subsystem/wheel1/wheel acceleration ==
  data: tau_axle input; alpha_w output; tau_brake input; I_in input; I_w input; r_w input; F_x input
function alpha_w = fcn(tau_axle, tau_brake, I_in, I_w, r_w, F_x)

alpha_w = (tau_axle - tau_brake - F_x * r_w) / (I_in + I_w);

== matlab function p4_individual_simulink/Driver/MATLAB Function5 ==
  data: X input; e output; Y input; psi input; x_vals input; y_vals input
function e = error(X, Y, psi, x_vals, y_vals)
%calculate the error for straights and curves
%straights
    e = 0;
    car_loc = [X, Y];
    trac = [x_vals, y_vals];
    dist=[];

    for i = 1:length(y_vals)
        dist(end+1) = ((trac(i,1)-car_loc(1))^2 + (trac(i,2) - car_loc(2))^2)^(1/2);
    end

    [~, idx] = min(dist);
    idx = idx+10;

    if idx > length(y_vals)
        idx = length(y_vals);
    end


    target = trac(idx,:);

    e = atan2(target(2)-car_loc(2), target(1)-car_loc(1)) - psi;
end

== matlab function p4_individual_simulink/CarBidyFrame2InertialFrame/KinematicVehicleModel ==
  data: vx input; vy input; Xdot output; psi input; Ydot output
function [Xdot, Ydot] = fcn(vx, vy, psi)
    temp = TF(psi) * [vx;vy];
    Xdot=temp(1);
    Ydot=temp(2);
end

function y = TF(psi)
    y= [cos(psi), -sin(psi); sin(psi),cos(psi)];
end

== matlab function p4_individual_simulink/Driver/MATLAB Function ==
  data: alpha output; diff input; X input
function alpha = fcn(diff, X)

PID = 0.08;
alpha = abs(PID * diff);

end

== matlab function p4_individual_simulink/Driver/MATLAB Function1 ==
  data: alpha input; throttle output; brake output
function [throttle, brake] = fcn(alpha)
    if alpha >= 0 
        throttle = alpha;
        brake = 0;
    elseif alpha < 0
        throttle = 0;
        brake = alpha;
    else
        throttle = alpha;
        brake = 0;
    end

== matlab function p4_individual_simulink/Subsystem1/Subsystem/wheel1/MATLAB Function ==
  data: lambda input; F_x output; lambda_max input; normal_stiffness input; mu input; mass input
function F_x = tire_tractive_force(lambda, lambda_max, normal_stiffness, mu, mass)

g = 9.81; %m/s^2 gravity
N = mass * g/4; %normal force on all 4 tires
C_lambda = normal_stiffness * mu * N;

if lambda >= 0
    F_x = C_lambda * min(lambda_max, lambda);
else
    F_x = C_lambda * max(-lambda_max, lambda);
end

== matlab function p4_individual_simulink/Driver/MATLAB Function3 ==
  data: regen input; brake output; actual_speed input
function brake = fcn(regen, actual_speed)

brake = regen*actual_speed;

end

== matlab function p4_individual_simulink/Subsystem1/Subsystem/Electric Motor Drve/Battery/Battery ==
  data: I_bat input; batt_mod output; SOC input
function batt_mod = fcn(I_bat, SOC)
    if SOC <=.1
        batt_mod = 0;
    else
        batt_mod = I_bat;
    end

== matlab function p4_individual_simulink/Subsystem1/Subsystem/Electric Motor Drve/Electric Motor/MATLAB Function ==
  data: Tm input; I_bus output; Wm input; Effm input; V_bus input; Pe output
function [I_bus, Pe] = fcn(Tm, Wm, Effm, V_bus)
    Pm = Tm*Wm;
    sgn_M = Pm / (abs(Pm) + 0.001);
    Pe = Pm / (Effm^sgn_M);
    if V_bus > 1
        I_bus = Pe/V_bus;
    else
        I_bus = 0;
    end

== matlab function p4_individual_simulink/Driver/MATLAB Function4 ==
  data: deltaf output; vx input; lr input; lf input; PID input
function deltaf = fcn(vx, lr, lf, PID)

    L = lr + lf;
    psi_dot = 2*vx*sin(PID)/L;
    deltaf = psi_dot;
end
